simulink model "velo_id_verify_simu"  (R2020b)
settings: Solver=VariableStepAuto  StartTime=0.0  StopTime=20  RelTol=1e-3
values from neighbouring files (symbols this model uses):
  K = 0.760983012589    [model_data.mat]    (also in velo_id_verify.m = K_id; velo_modern_con.m = K_id; velo_modon_con.m = K_id; velo_pi_mbd.m = K_id)
  p_const = 0.7    [velo_id_gain.m]    (also in velo_id_gain_tc.m = 0.5; velo_id_tc.m = 0.5; velo_id_verify.m = 1; velo_pi_mbd.m = 1)
  r_const = 0.7    [velo_id_gain.m]    (also in velo_id_gain_tc.m = 1.3; velo_id_tc.m = 1.3; velo_id_verify.m = 0.75)
  s_time = 10    [velo_id_gain.m]    (also in velo_id_gain_tc.m; velo_id_tc.m; velo_id_verify.m; velo_pi_mbd.m = 5)
  T = 0.44    [model_data.mat]    (also in velo_id_verify.m = T_id; velo_modern_con.m = T_id; velo_modon_con.m = T_id; velo_pi_mbd.m = T_id)
  u_offset = 0.280493571056    [model_data.mat]    (also in velo_id_gain.m = -P(2)/P(1); velo_id_gain_tc.m = (K_id*r_const-c1)/K_id; velo_id_tc.m = (K_id*r_const-c1)/K_id; velo_modern_con.m = u_offset)
libraries: arduino_io_lib x4
settings Model: Creator=kei55  LastModifiedBy=kei55

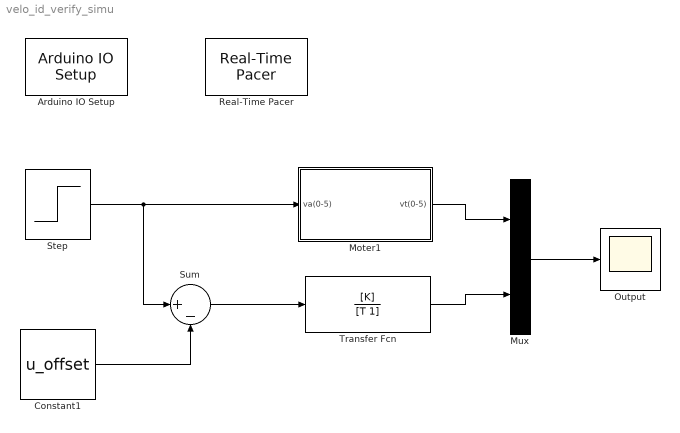
== system velo_id_verify_simu ==
  Arduino IO Setup : arduino_io_lib/Arduino IO Setup  Priority=3  arduinoVar=Temporary arduino variable: Arduino1  workspaceVarName=a  comPort=COM3
  Constant1 : Constant  Value=u_offset
  Moter1 : Subsystem
  Mux : Mux  Inputs=2
  Output : Scope
  Real-Time Pacer : arduino_io_lib/Real-Time Pacer  simTimePerRealTime=1
  Step : Step  Time=s_time  Before=r_const  After=r_const+p_const  SampleTime=0
  Sum : Sum  Inputs=|+-
  Transfer Fcn : TransferFcn  Numerator=[K]  Denominator=[T 1]
  wires:
  Mux/1 -> Output/1
  Moter1/1(vt(0-5)) -> Mux/1
  Step/1 -> Moter1/1(va(0-5)), Sum/1
  Constant1/1 -> Sum/2
  Sum/1 -> Transfer Fcn/1
  Transfer Fcn/1 -> Mux/2

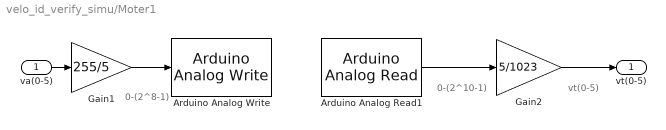
== system velo_id_verify_simu/Moter1 ==
  note: 0-(2^8-1)
  note: 0-(2^10-1)
  note: vt(0-5)
  va(0-5) : Inport
  Arduino Analog Read1 : arduino_io_lib/Arduino Analog Read  arduinoVar=Temporary arduino variable: Arduino1  arduinoPin=0  T=1/50
  Arduino Analog Write : arduino_io_lib/Arduino Analog Write  arduinoVar=Temporary arduino variable: Arduino1  arduinoPin=3  T=1/50
  Gain1 : Gain  Gain=255/5
  Gain2 : Gain  Gain=5/1023
  vt(0-5) : Outport
  wires:
  Arduino Analog Read1/1 -> Gain2/1
  Gain1/1 -> Arduino Analog Write/1
  Gain2/1 -> vt(0-5)/1
  va(0-5)/1 -> Gain1/1
